simulink model "DEF_2GFL_Eugenie"  (R2022b)
settings: Solver=FixedStepAuto  StartTime=0  StopTime=10  FixedStep=Ts  RelTol=1e-3
undefined symbols (not defined in the file or in its folder): ApparatusDiscreDamping, ApparatusPara, ApparatusPowerFlow, ApparatusType, OtherInputs, PowerFlow, Sbase, Ts, Vbase, Wbase, x_e, Ybase, Zbase
libraries: SimplusGT x10, spsGroundLib x5, spsThreePhaseSeriesRLCBranchLib x4, spsSawtoothGeneratorLib x4, spsabctoAlphaBetaZeroLib x4, spsControlledCurrentSourceLib x3, spsCurrentMeasurementLib x3, spsVoltageMeasurementLib x3, spsThreePhaseParallelRLCBranchLib x2, sps_lib x1
(part 2 of 2)

== system DEF_2GFL_Eugenie/VSI-PLL2/Forced oscillation2 ==
  angr : Inport
  Constant : Constant
  Divide : Product  Inputs=**
  Divide1 : Product  Inputs=**
  Gain4 : Gain  Gain=0
  Sine Wave : Sin  Frequency=2*pi*3  Phase=pi  SampleTime=0
  Step : Step  Time=2  SampleTime=0
  Out1 : Outport
  wires:
  Gain4/1 -> Divide/1
  Divide1/1 -> Out1/1
  Divide/1 -> Divide1/1
  Step/1 -> Divide1/2
  Sine Wave/1 -> Divide/2
  Constant/1 -> Gain4/1

== system DEF_2GFL_Eugenie/VSI-PLL2/Forced oscillation3 ==
  theta : Inport
  Divide : Product  Inputs=**
  Divide1 : Product  Inputs=**
  Gain4 : Gain  Gain=0
  Sine Wave : Sin  Frequency=2*pi*3  SampleTime=0
  Step : Step  Time=2  SampleTime=0
  Out1 : Outport
  wires:
  theta/1 -> Gain4/1
  Sine Wave/1 -> Divide/2
  Step/1 -> Divide1/2
  Divide/1 -> Divide1/1
  Divide1/1 -> Out1/1
  Gain4/1 -> Divide/1

== system DEF_2GFL_Eugenie/VSI-PLL2/Forced oscillation4 ==
  id : Inport
  Divide : Product  Inputs=**
  Divide1 : Product  Inputs=**
  Gain4 : Gain  Gain=0
  Sine Wave : Sin  Frequency=2*pi*3  Phase=180  SampleTime=0
  Step : Step  Time=2  SampleTime=0
  Out1 : Outport
  wires:
  Gain4/1 -> Divide/1
  Divide1/1 -> Out1/1
  Divide/1 -> Divide1/1
  Step/1 -> Divide1/2
  Sine Wave/1 -> Divide/2
  id/1 -> Gain4/1

== system DEF_2GFL_Eugenie/VSI-PLL2/Forced oscillation5 ==
  iq : Inport
  Divide : Product  Inputs=**
  Divide1 : Product  Inputs=**
  Gain4 : Gain  Gain=0
  Sine Wave : Sin  Frequency=2*pi*3  SampleTime=0
  Step : Step  Time=2  SampleTime=0
  Out1 : Outport
  wires:
  iq/1 -> Gain4/1
  Sine Wave/1 -> Divide/2
  Step/1 -> Divide1/2
  Divide/1 -> Divide1/1
  Divide1/1 -> Out1/1
  Gain4/1 -> Divide/1

== system DEF_2GFL_Eugenie/VSI-PLL2/PQ Calculation (dq-Frame)1 ==
  note: Power calculation.
      |
      | Author(s): Yitong Li
      |
      | Notes:
      |
      | The calculation is done in dq frame.
  vdq : Inport
  idq : Inport  Port=2
  Mux : Mux  Inputs=2
  Mux1 : Mux  Inputs=2
  P = vd*id+vq*iq : Fcn  Expr=u[1]*u[3]+u[2]*u[4]
  Q = -vd*iq+vq*id : Fcn  Expr=-u[1]*u[4]+u[2]*u[3]
  pq : Outport
  wires:
  Mux/1 -> pq/1
  P = vd*id+vq*iq/1 -> Mux/1
  vdq/1 -> Mux1/1
  idq/1 -> Mux1/2
  Mux1/1 -> P = vd*id+vq*iq/1, Q = -vd*iq+vq*id/1
  Q = -vd*iq+vq*id/1 -> Mux/2

== system DEF_2GFL_Eugenie/VSI-PLL2/abc -> dq (Power-Invariant)1 ==
  note: Frame transformation from abc to dq.
      |
      | Author(s): Yitong Li
      |
      | Notes:
      |
      | The transformation is power-invariant.
      |
      | theta is the angle that d axis leads a axis.
      |
      | q axis leads d axis by 90 degrees.
  abc : Inport
  theta : Inport  Port=2
  ->d : Fcn  Expr=cos(u(4))*u(1) + cos(u(4)-2/3*pi)*u(2) + cos(u(4)-4/3*pi)*u(3)
  ->q : Fcn  Expr=-sin(u(4))*u(1) - sin(u(4)-2/3*pi)*u(2) - sin(u(4)-4/3*pi)*u(3)
  Gain : Gain  Gain=sqrt(2/3)
  Mux5 : Mux  Inputs=2
  Mux6 : Mux  Inputs=2
  dq : Outport
  wires:
  abc/1 -> Gain/1
  ->d/1 -> Mux6/1
  Gain/1 -> Mux5/1
  theta/1 -> Mux5/2
  ->q/1 -> Mux6/2
  Mux6/1 -> dq/1
  Mux5/1 -> ->d/1, ->q/1

== system DEF_2GFL_Eugenie/VSI-PLL2/abc -> dq (Power-Invariant)2 ==
  note: Frame transformation from abc to dq.
      |
      | Author(s): Yitong Li
      |
      | Notes:
      |
      | The transformation is power-invariant.
      |
      | theta is the angle that d axis leads a axis.
      |
      | q axis leads d axis by 90 degrees.
  abc : Inport
  theta : Inport  Port=2
  ->d : Fcn  Expr=cos(u(4))*u(1) + cos(u(4)-2/3*pi)*u(2) + cos(u(4)-4/3*pi)*u(3)
  ->q : Fcn  Expr=-sin(u(4))*u(1) - sin(u(4)-2/3*pi)*u(2) - sin(u(4)-4/3*pi)*u(3)
  Gain : Gain  Gain=sqrt(2/3)
  Mux5 : Mux  Inputs=2
  Mux6 : Mux  Inputs=2
  dq : Outport
  wires:
  abc/1 -> Gain/1
  ->d/1 -> Mux6/1
  Gain/1 -> Mux5/1
  theta/1 -> Mux5/2
  ->q/1 -> Mux6/2
  Mux6/1 -> dq/1
  Mux5/1 -> ->d/1, ->q/1

== system DEF_2GFL_Eugenie/VSI-PLL2/dq -> abc (Power-Invariant)1 ==
  note: Frame transformation from dq to abc.
      |
      | Author(s): Yitong Li
      |
      | Notes:
      |
      | The transformation is power-invariant.
      |
      | theta is the angle that dq axis leads alpha/beta axis, specifically, d axis leads alpha axis.
  dq : Inport
  theta : Inport  Port=2
  ->a : Fcn  Expr=cos(u(3))*u(1) - sin(u(3))*u(2)
  ->b : Fcn  Expr=cos(u(3)-2/3*pi)*u(1) - sin(u(3)-2/3*pi)*u(2)
  ->c : Fcn  Expr=cos(u(3)-4/3*pi)*u(1) - sin(u(3)-4/3*pi)*u(2)
  Gain : Gain  Gain=sqrt(2/3)
  Mux5 : Mux  Inputs=2
  Mux6 : Mux  Inputs=3
  abc : Outport
  wires:
  ->b/1 -> Mux6/2
  ->a/1 -> Mux6/1
  Gain/1 -> Mux5/1
  dq/1 -> Gain/1
  ->c/1 -> Mux6/3
  Mux6/1 -> abc/1
  Mux5/1 -> ->b/1, ->a/1, ->c/1
  theta/1 -> Mux5/2

== system DEF_2GFL_Eugenie/DEF_DQ_Fan/DEF_DualFrictionFan2/Initial_filter2 ==
  original : Inport
  Clock1 : Clock
  Gain7 : Gain
  Gain8 : Gain  Gain=0
  Switch3 : Switch  Criteria=u2 > Threshold  Threshold=1.5  SaturateOnIntegerOverflow=off  InputSameDT=off
  filtered : Outport
  wires:
  Switch3/1 -> filtered/1  "d"
  original/1 -> Gain8/1, Gain7/1
  Gain7/1 -> Switch3/1
  Gain8/1 -> Switch3/3
  Clock1/1 -> Switch3/2

== system DEF_2GFL_Eugenie/DEF_DQ_Fan/DEF_DualFrictionFan2/Initial_filter4 ==
  original : Inport
  Clock1 : Clock
  Gain7 : Gain
  Gain8 : Gain  Gain=0
  Switch3 : Switch  Criteria=u2 > Threshold  Threshold=1.5  SaturateOnIntegerOverflow=off  InputSameDT=off
  filtered : Outport
  wires:
  Clock1/1 -> Switch3/2
  Gain8/1 -> Switch3/3
  Gain7/1 -> Switch3/1
  original/1 -> Gain7/1, Gain8/1
  Switch3/1 -> filtered/1  "d"

== system DEF_2GFL_Eugenie/DEF_DQ_Fan/dq2DQ/Triggered Subsystem1 ==
  a : Inport
  b : Inport  Port=2
  Trigger : TriggerPort  VariantControl=(inherit)
  Sum : Sum  Inputs=|+-
  a-b : Outport  InitialOutput=0
  wires:
  Sum/1 -> a-b/1
  b/1 -> Sum/2
  a/1 -> Sum/1

== system DEF_2GFL_Eugenie/DEF_DQ_Fan/dq2DQ1/Triggered Subsystem1 ==
  a : Inport
  b : Inport  Port=2
  Trigger : TriggerPort  VariantControl=(inherit)
  Sum : Sum  Inputs=|+-
  a-b : Outport  InitialOutput=0
  wires:
  a/1 -> Sum/1
  b/1 -> Sum/2
  Sum/1 -> a-b/1

== system DEF_2GFL_Eugenie/DEF_DQ_Fan1/DEF_DualFrictionFan2/Initial_filter2 ==
  original : Inport
  Clock1 : Clock
  Gain7 : Gain
  Gain8 : Gain  Gain=0
  Switch3 : Switch  Criteria=u2 > Threshold  Threshold=1.5  SaturateOnIntegerOverflow=off  InputSameDT=off
  filtered : Outport
  wires:
  Clock1/1 -> Switch3/2
  Gain8/1 -> Switch3/3
  Gain7/1 -> Switch3/1
  original/1 -> Gain7/1, Gain8/1
  Switch3/1 -> filtered/1  "d"

== system DEF_2GFL_Eugenie/DEF_DQ_Fan1/DEF_DualFrictionFan2/Initial_filter4 ==
  original : Inport
  Clock1 : Clock
  Gain7 : Gain
  Gain8 : Gain  Gain=0
  Switch3 : Switch  Criteria=u2 > Threshold  Threshold=1.5  SaturateOnIntegerOverflow=off  InputSameDT=off
  filtered : Outport
  wires:
  Switch3/1 -> filtered/1  "d"
  original/1 -> Gain8/1, Gain7/1
  Gain7/1 -> Switch3/1
  Gain8/1 -> Switch3/3
  Clock1/1 -> Switch3/2

== system DEF_2GFL_Eugenie/DEF_DQ_Fan1/dq2DQ/Triggered Subsystem1 ==
  a : Inport
  b : Inport  Port=2
  Trigger : TriggerPort  VariantControl=(inherit)
  Sum : Sum  Inputs=|+-
  a-b : Outport  InitialOutput=0
  wires:
  a/1 -> Sum/1
  b/1 -> Sum/2
  Sum/1 -> a-b/1

== system DEF_2GFL_Eugenie/DEF_DQ_Fan1/dq2DQ1/Triggered Subsystem1 ==
  a : Inport
  b : Inport  Port=2
  Trigger : TriggerPort  VariantControl=(inherit)
  Sum : Sum  Inputs=|+-
  a-b : Outport  InitialOutput=0
  wires:
  Sum/1 -> a-b/1
  b/1 -> Sum/2
  a/1 -> Sum/1
